simulink model "filter8tap"  (Simulink 6.3)
settings: Solver=ode45  StartTime=0.0  StopTime=100.0  RelTol=1e-3
InitFcn:
  | %% DSPBuilder Start
  | alt_dspbuilder_update_model(bdroot)
  | %% DSPBuilder End
libraries: allblocks_alteradspbuilder2 x4
settings Model: Creator=gnixon  LastModifiedBy=delphick
settings DataIOCC: SignalLoggingName=sigsOut
settings DebuggingCC: SolverPrmCheckMsg=none
settings HardwareCC: TargetUnknown=on
settings GRTTargetCC: ModelReferenceCompliant=off  MatFileLogging=off

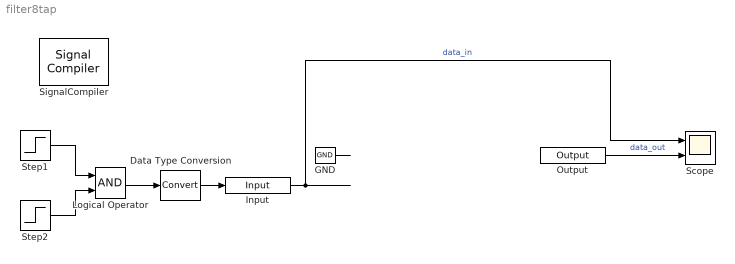
== system filter8tap ==
  Data Type Conversion : DataTypeConversion  OutDataTypeMode=double  SaturateOnIntegerOverflow=on  RndMeth=Zero
  GND : allblocks_alteradspbuilder2/GND  SpecifyClock=off
  Input : allblocks_alteradspbuilder2/Input  iofile=C:\workspace_clean\Documentation\DesignExamples\Tutorials\BlackBox\SubSystemBuilder\tb_filter8tap\filter8tap_Input.salt  BusType=Signed Integer  bwl=16  bwr=0  SpecifyClock=off  PORTTYPE=Input
  Logical Operator : Logic  AllPortsSameDT=off
  Output : allblocks_alteradspbuilder2/Output  iofile=C:\workspace_clean\Documentation\DesignExamples\Tutorials\BlackBox\SubSystemBuilder\tb_filter8tap\filter8tap_Output.capture  BusType=Signed Integer  bwl=33  bwr=0  PORTTYPE=Output
  Scope : Scope  NumInputPorts=2
      settings: YMin=-5~-5  YMax=5~5
  SignalCompiler : allblocks_alteradspbuilder2/Signal Compiler  DeviceFamily=Stratix III  DeviceName=AUTO  EnableSignalTap=off  SignalTapDepth=128  UseBoardBlock=off  StpUseDefaultClock=on  StpClock=clock
  Step1 : Step  Time=10  SampleTime=1
  Step2 : Step  Time=11  Before=1  After=0  SampleTime=1
  wires:
  Step1/1 -> Logical Operator/1
  Step2/1 -> Logical Operator/2
  Logical Operator/1 -> Data Type Conversion/1
  GND/1 -> ?
  Input/1 -> Scope/1  "data_in"
  ? -> Output/1
  Output/1 -> Scope/2  "data_out"
  Data Type Conversion/1 -> Input/1
